simulink model "PubIfDecisionLSM_MDL"  (R2020b)
settings: configuration reference "DspaceConfig" (kept outside this file)
PostLoadFcn:
  | if any(exist('dsrtsu_mdlpostloadfcn', 'file') ~= 0), dsrtsu_mdlpostloadfcn('Execute', bdroot); end
InitFcn:
  | , if any(exist('rtifpga_mdlclblib', 'file') ~= 0), rtifpga_mdlclblib('Init', bdroot); end,
  | , if any(exist('dsmpb_private', 'file') ~= 0), dsmpb_private('dsmpb_mdlclblib', 'Init', bdroot); end,
values from neighbouring files (symbols this model uses):
  P_LSM_ALC_Enable = 0.0    [LSM_Parameter.sldd]
  P_LSM_AwayEdge_offset = 0.1    [LSM_Parameter.sldd]
  P_LSM_CentValidErr = 1.0    [LSM_Parameter.sldd]
  P_LSM_DOP_C0_EN_Limit = 0.8    [LSM_Parameter.sldd]
  P_LSM_DOP_C0_out_Limit = 2.0    [LSM_Parameter.sldd]
  P_LSM_DOP_C1_EN_Limit : value not decoded    [LSM_Parameter.sldd]
  P_LSM_DOP_C1_out_Limit : value not decoded    [LSM_Parameter.sldd]
  P_LSM_DOP_C1AndC2_Lim_X : value not decoded    [LSM_Parameter.sldd]
  P_LSM_DOP_C2_EN_Limit : value not decoded    [LSM_Parameter.sldd]
  P_LSM_DOP_C2_out_Limit : value not decoded    [LSM_Parameter.sldd]
  P_LSM_DOP_In_Pre2Dop_Dis = 1.0    [LSM_Parameter.sldd]
  P_LSM_DOP_Out_Pre2Dop_Dis = 2.0    [LSM_Parameter.sldd]
  P_LSM_DOP_PreDis_X : value not decoded    [LSM_Parameter.sldd]
  P_LSM_DOP_PreDis_Y : value not decoded    [LSM_Parameter.sldd]
  P_LSM_DOPEnableSW = 1.0    [LSM_Parameter.sldd]
  P_LSM_DOPValid_CheckTime = 0.06    [LSM_Parameter.sldd]
  P_LSM_DoubleLine_Curr2Cent_Dislimit = 0.5    [LSM_Parameter.sldd]
  P_LSM_DoubleLine_Dop2Cent_Dislimit = 0.5    [LSM_Parameter.sldd]
  P_LSM_DoubleLine_DOPOut_C1 : value not decoded    [LSM_Parameter.sldd]
  P_LSM_DoubleLine_Pre2Cent_Dislimit = 1.0    [LSM_Parameter.sldd]
  P_LSM_Error_Limit = 0.5    [LSM_Parameter.sldd]
  P_LSM_IFV2CenterAxis = 0.0    [LSM_Parameter.sldd]
  P_LSM_IFV2RearAxis = 0.0    [LSM_Parameter.sldd]
  P_LSM_Line2Edge_limit = 0.5    [LSM_Parameter.sldd]
  P_LSM_Line_Error = 0.1    [LSM_Parameter.sldd]
  P_LSM_LineSTD_Limit = 0.15    [LSM_Parameter.sldd]
  P_LSM_NOH_Switch = 0.0    [LSM_Parameter.sldd]
  P_LSM_OTL_C0_Factor = 1.0    [LSM_Parameter.sldd]
  P_LSM_OTL_C1_Factor = 0.5    [LSM_Parameter.sldd]
  P_LSM_OTL_C2_Factor = 0.5    [LSM_Parameter.sldd]
  P_LSM_Pre2OnlyLineDis = 5.0    [LSM_Parameter.sldd]
  P_LSM_Pre_t = 0.0    [LSM_Parameter.sldd]
  P_LSM_SingleLine_Cent2Edge_Dislimit = 100.0    [LSM_Parameter.sldd]
  P_LSM_SingleLine_Curr2Cent_Dislimit = 0.2    [LSM_Parameter.sldd]
  P_LSM_SingleLine_Dop2Cent_Dislimit = 0.2    [LSM_Parameter.sldd]
  P_LSM_SingleLine_DOPOut_C1 : value not decoded    [LSM_Parameter.sldd]
  P_LSM_SingleLine_Pre2Cent_Dislimit = 0.5    [LSM_Parameter.sldd]
  P_LSM_TJALimitSpd = 60.0    [LSM_Parameter.sldd]
undefined symbols (not defined in the file or in its folder): P_lCS_IFV2CenterAxis, P_LCS_IFV2RearAxis, P_LSM_EntryEdge_offset, P_LSM_EntryLnChngEnSwitch, P_LSM_EntryVanishDis, P_LSM_LinetLostTime, P_LSM_LineWijCal_C12, P_LSM_LineWijCal_C13, P_LSM_MapValid_ErrorSwitch, P_LSM_PosLineLcFac, P_LSM_SpdLim_Stub_Spd, P_LSM_SpdLim_StubLength, P_LSM_SpdTurnAlarm
libraries: simulink x324, TrueDurationTime x11
(part 11 of 25)

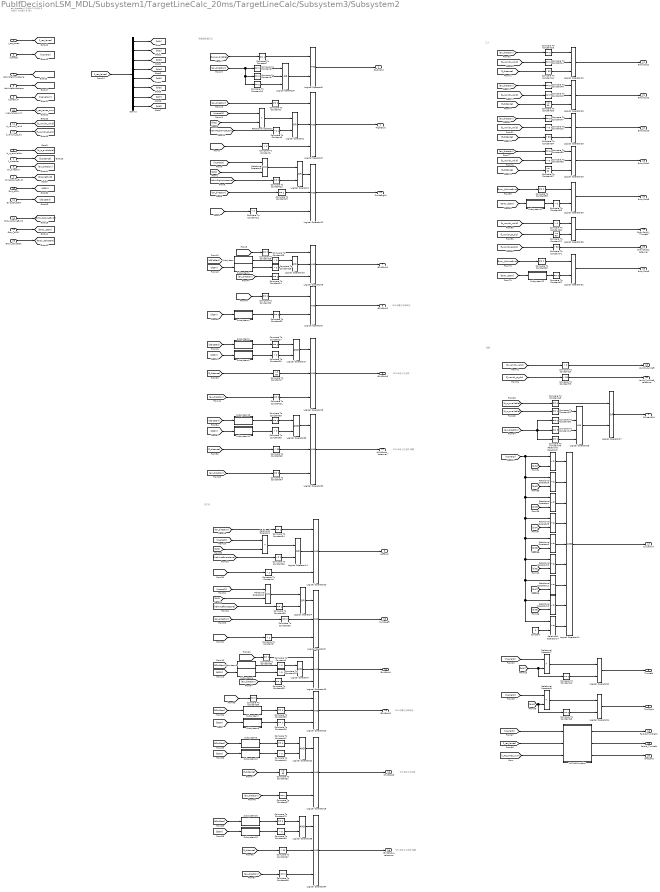
== system PubIfDecisionLSM_MDL/Subsystem1/TargetLineCalc_20ms/TargetLineCalc/Subsystem3/Subsystem2 ==
  note: 左汇出
  note: 巡航
  note: 汇入
  note: %%未走上汇出线
  note: %%沿着汇出线驶出
  note: %%未走上汇出线
  note: en_direction
      | 1 左驶出
      | 2 右驶出
      | 3 左直行
      | 4 右直行
      | 5 驶入
  note: %%沿着汇出线驶出
  note: 高速或匝道汇出
  note: %%未走上汇出线,接管
  note: %%未走上汇出线,接管
  Exit_bIsLineExist : Inport
  f_distance : Inport  Port=2
  b_is_available : Inport  Port=3
  i_rec_lanes : Inport  Port=4
  nLaneID : Inport  Port=5
  en_direction : Inport  Port=6
  VehInRightmostLane : Inport  Port=7  OutDataTypeStr=boolean
  VehInLeftmostLane : Inport  Port=8  OutDataTypeStr=boolean
  nLaneNum : Inport  Port=9
  i_rec_lanes_num : Inport  Port=10
  " b_vanish_valid" : Inport  Port=11
  " Exit_dDisStart" : Inport  Port=12
  Exit_dC0V : Inport  Port=13
  Entry_bIsLineExist : Inport  Port=14
  Entry_dDisStart : Inport  Port=15
  Entry_dC0V : Inport  Port=16
  " f_vanish_pt_dis " : Inport  Port=17
  Compare To Constant{1,4..5,12} (4 alike) : simulink/Logic and Bit Operations/Compare To Constant  relop=<  const=2  OutDataTypeStr=boolean
  Compare To Constant{10,16,46..47,56} (5 alike) : simulink/Logic and Bit Operations/Compare To Constant  relop===  const=5  OutDataTypeStr=boolean
  Compare To Constant11 : simulink/Logic and Bit Operations/Compare To Constant  relop===  const=3  OutDataTypeStr=boolean
  Compare To Constant{6,13,15,20,25..26,29,40,55,59,62,66,69} (13 alike) : simulink/Logic and Bit Operations/Compare To Constant  relop=>  const=0  OutDataTypeStr=boolean
  Compare To Constant{14,27..28,30,41,45,48,50,52,61,65,70} (12 alike) : simulink/Logic and Bit Operations/Compare To Constant  relop===  const=0  OutDataTypeStr=boolean
  Compare To Constant17 : simulink/Logic and Bit Operations/Compare To Constant  relop=>=  const=50  OutDataTypeStr=boolean
  Compare To Constant{2,9,18..19,21,23..24,32,38,58,60,64} (12 alike) : simulink/Logic and Bit Operations/Compare To Constant  relop===  const=2  OutDataTypeStr=boolean
  Compare To Constant{7..8,22,33..35,37,39,51,68} (10 alike) : simulink/Logic and Bit Operations/Compare To Constant  relop===  const=1  OutDataTypeStr=boolean
  Compare To Constant3 : simulink/Logic and Bit Operations/Compare To Constant  relop=~=  const=1  OutDataTypeStr=boolean
  Compare To Constant31 : simulink/Logic and Bit Operations/Compare To Constant  relop=>=  const=50  OutDataTypeStr=boolean
  Compare To Constant36 : simulink/Logic and Bit Operations/Compare To Constant  relop=~=  const=1  OutDataTypeStr=boolean
  Compare To Constant42 : simulink/Logic and Bit Operations/Compare To Constant  relop=~=  const=0  OutDataTypeStr=boolean
  Compare To Constant43 : simulink/Logic and Bit Operations/Compare To Constant  relop=~=  const=0  OutDataTypeStr=boolean
  Compare To Constant44 : simulink/Logic and Bit Operations/Compare To Constant  relop=>  const=50  OutDataTypeStr=boolean
  Compare To Constant49 : simulink/Logic and Bit Operations/Compare To Constant  relop===  const=4  OutDataTypeStr=boolean
  Compare To Constant53 : simulink/Logic and Bit Operations/Compare To Constant  relop=<=  const=50  OutDataTypeStr=boolean
  Compare To Constant54 : simulink/Logic and Bit Operations/Compare To Constant  relop=>  const=50  OutDataTypeStr=boolean
  Compare To Constant57 : simulink/Logic and Bit Operations/Compare To Constant  relop=<=  const=50  OutDataTypeStr=boolean
  Compare To Constant{63,67,71,73} (4 alike) : simulink/Logic and Bit Operations/Compare To Constant  relop=<  const=50  OutDataTypeStr=boolean
  Compare To Constant72 : simulink/Logic and Bit Operations/Compare To Constant  relop=>=  const=50  OutDataTypeStr=boolean
  Constant : Constant  Value=0  OutDataTypeStr=uint8
  Demux : Demux  Outputs=8
  Logical Operator{1..2,4,14,27} (5 alike) : Logic  Operator=OR  AllPortsSameDT=off  OutDataTypeStr=boolean
  Logical Operator{3,5,10,12..13,15,18..20,23,25..26,29,32,34} (15 alike) : Logic  Inputs=3  AllPortsSameDT=off  OutDataTypeStr=boolean
  Logical Operator11 : Logic  Inputs=9'  AllPortsSameDT=off  OutDataTypeStr=boolean
  Logical Operator{6..8,16..17,21..22,24,30..31,33,35..36} (13 alike) : Logic  AllPortsSameDT=off  OutDataTypeStr=boolean
  Logical Operator28 : Logic  Inputs=4  AllPortsSameDT=off  OutDataTypeStr=boolean
  Logical Operator9 : Logic  Operator=OR  Inputs=3  AllPortsSameDT=off  OutDataTypeStr=boolean
  MATLAB Function : MATLAB Function  TreatAsAtomicUnit=on
  Relational Operator : RelationalOperator  Operator=<  OutDataTypeStr=boolean  RndMeth=Simplest
  Relational Operator1 : RelationalOperator  Operator=>  OutDataTypeStr=boolean  RndMeth=Simplest
  Relational Operator{2..6,10,12..14} (9 alike) : RelationalOperator  Operator=~=  OutDataTypeStr=boolean  RndMeth=Simplest
  Relational Operator11 : RelationalOperator  Operator===  OutDataTypeStr=boolean  RndMeth=Simplest
  Relational Operator7 : RelationalOperator  Operator=>  OutDataTypeStr=boolean  RndMeth=Simplest
  Relational Operator8 : RelationalOperator  Operator=<  OutDataTypeStr=boolean  RndMeth=Simplest
  Relational Operator9 : RelationalOperator  Operator===  OutDataTypeStr=boolean  RndMeth=Simplest
  Subsystem : Subsystem
  Subsystem1 : Subsystem
  Subsystem10 : Subsystem
  Subsystem11 : Subsystem
  Subsystem12 : Subsystem
  Subsystem13 : Subsystem
  Subsystem14 : Subsystem
  Subsystem15 : Subsystem
  Subsystem16 : Subsystem
  Subsystem2 : Subsystem
  Subsystem3 : Subsystem
  Subsystem4 : Subsystem
  Subsystem5 : Subsystem
  Subsystem6 : Subsystem
  Subsystem7 : Subsystem
  Subsystem8 : Subsystem
  Subsystem9 : Subsystem
  StubValid : Outport
  RightStub : Outport  Port=2
  LeftStub : Outport  Port=3
  CruiseValid : Outport  Port=4
  TurnLeft : Outport  Port=5
  TurnRight : Outport  Port=6
  rExitStub1 : Outport  Port=7
  rExitStub2 : Outport  Port=8
  rExitStub3 : Outport  Port=9
  Vanish_turnleft : Outport  Port=10
  EntryStub1 : Outport  Port=11
  CruiseRight : Outport  Port=12
  CruiseLeft : Outport  Port=13
  lExitStub1 : Outport  Port=14
  lExitStub2 : Outport  Port=15
  lExitStub3 : Outport  Port=16
  CruiseTurn : Outport  Port=17
  Forbid_TurnRight : Outport  Port=18
  Forbid_TurnLeft : Outport  Port=19
  OneLane : Outport  Port=20
  EntryStub2 : Outport  Port=21
  EntryStub3 : Outport  Port=22
  EntryStub4 : Outport  Port=23
  EntryStub5 : Outport  Port=24
  EntryStub6 : Outport  Port=25
  EntryStub5_TurnLeft : Outport  Port=26
  rExitStub4_takeover : Outport  Port=27
  lExitStub4_takeover : Outport  Port=28
  EntryStub5_takeover : Outport  Port=29
  Vanish_turnleft_takeover : Outport  Port=30
  wires:
  Compare To Constant40/1 -> Logical Operator22/2
  Compare To Constant41/1 -> Logical Operator22/1
  Subsystem9/1(y) -> Compare To Constant41/1
  [dDisStart] -> Subsystem9/1(u)
  [dC0V] -> Subsystem10/1(u)
  Subsystem10/1(y) -> Compare To Constant40/1
  Subsystem8/1(y) -> Compare To Constant28/1
  [dC0V] -> Subsystem8/1(u)
  [dDisStart] -> Subsystem7/1(u)
  Subsystem7/1(y) -> Compare To Constant30/1
  Compare To Constant30/1 -> Logical Operator23/2
  Compare To Constant28/1 -> Logical Operator23/3
  Logical Operator7/1 -> Logical Operator19/2
  Compare To Constant13/1 -> Logical Operator7/2
  Compare To Constant6/1 -> Logical Operator7/1
  Subsystem5/1(y) -> Compare To Constant6/1
  [dDisStart] -> Subsystem5/1(u)
  [dC0V] -> Subsystem6/1(u)
  Subsystem6/1(y) -> Compare To Constant13/1
  Subsystem3/1(y) -> Compare To Constant29/1
  [dC0V] -> Subsystem3/1(u)
  [dDisStart] -> Subsystem2/1(u)
  Subsystem2/1(y) -> Compare To Constant27/1
  Compare To Constant27/1 -> Logical Operator17/1
  Compare To Constant29/1 -> Logical Operator17/2
  Compare To Constant52/1 -> Logical Operator6/2
  [dC0V] -> Subsystem4/1(u)
  Subsystem4/1(y) -> Compare To Constant52/1
  Subsystem1/1(y) -> Compare To Constant26/1
  [dC0V] -> Subsystem1/1(u)
  [dDisStart] -> Subsystem/1(u)
  [i_rec_lanes_num] -> MATLAB Function/3(i_rec_lanes_num)
  MATLAB Function/3(OneLane) -> OneLane/1
  MATLAB Function/2(Forbid_TurnLeft) -> Forbid_TurnLeft/1
  MATLAB Function/1(Forbid_TurnRight) -> Forbid_TurnRight/1
  [nLaneID] -> MATLAB Function/1(nLaneID)
  [i_rec_lanes] -> MATLAB Function/2(i_rec_lanes)
  Logical Operator27/1 -> CruiseValid/1  "CruiseValid"
  Compare To Constant49/1 -> Logical Operator28/4
  Compare To Constant51/1 -> Logical Operator28/1
  [b_is_available] -> Compare To Constant51/1
  [en_direction] -> Compare To Constant11/1, Compare To Constant49/1, Compare To Constant50/1
  Compare To Constant50/1 -> Logical Operator28/2
  Compare To Constant11/1 -> Logical Operator28/3
  Logical Operator28/1 -> Logical Operator27/2
  Constant/1 -> Relational Operator14/2
  Relational Operator14/1 -> Logical Operator11/9
  Compare To Constant12/1 -> Logical Operator12/3
  Logical Operator8/1 -> StubValid/1  "StubValid"
  Logical Operator9/1 -> Logical Operator8/2
  Compare To Constant10/1 -> Logical Operator9/3
  Compare To Constant9/1 -> Logical Operator9/2
  Compare To Constant8/1 -> Logical Operator9/1
  [en_direction] -> Compare To Constant8/1, Compare To Constant9/1, Compare To Constant10/1
  Relational Operator7/1 -> Logical Operator21/1
  [bit8] -> Relational Operator13/2
  [bit7] -> Relational Operator12/2
  [bit6] -> Relational Operator10/2
  Relational Operator13/1 -> Logical Operator11/8
  Relational Operator12/1 -> Logical Operator11/7
  Relational Operator10/1 -> Logical Operator11/6
  [b_is_available] -> Compare To Constant48/1
  Compare To Constant48/1 -> Logical Operator27/1
  Compare To Constant37/1 -> Logical Operator18/3
  Logical Operator19/1 -> lExitStub1/1  "lExitStub1"
  [en_direction] -> Compare To Constant37/1
  Compare To Constant39/1 -> Logical Operator19/3
  [f_distance] -> Compare To Constant31/1
  [en_direction] -> Compare To Constant39/1
  Logical Operator18/1 -> lExitStub3/1  "lExitStub3"
  Logical Operator22/1 -> Logical Operator18/1
  Compare To Constant31/1 -> Logical Operator18/2
  [bIsLineExist] -> Compare To Constant32/1
  Compare To Constant32/1 -> Logical Operator19/1
  Compare To Constant38/1 -> Logical Operator23/1
  [bIsLineExist] -> Compare To Constant38/1
  Logical Operator23/1 -> lExitStub2/1  "lExitStub2"
  Logical Operator20/1 -> LeftStub/1  "LeftStub"
  [en_direction] -> Compare To Constant33/1  "LSM_Stub_Direction"
  Relational Operator1/1 -> Logical Operator14/1
  [bit1] -> Relational Operator1/2
  Logical Operator5/1 -> CruiseLeft/1  "CruiseLeft"
  [VehInLeftmostLane] -> Compare To Constant36/1
  Relational Operator11/1 -> Logical Operator4/1
  [nLaneID] -> Relational Operator1/1
  [VehInLeftmostLane] -> Compare To Constant35/1
  Compare To Constant35/1 -> Logical Operator4/2
  Logical Operator4/1 -> Logical Operator5/1
  Compare To Constant33/1 -> Logical Operator5/2
  [en_direction] -> Compare To Constant34/1  "LSM_Stub_Direction"
  Compare To Constant34/1 -> Logical Operator20/1
  [nLaneID] -> Relational Operator11/1
  [bit1] -> Relational Operator11/2
  Compare To Constant5/1 -> Logical Operator5/3
  Logical Operator14/1 -> Logical Operator20/2
  [bIsLineExist] -> Compare To Constant5/1
  Compare To Constant4/1 -> Logical Operator20/3
  [bIsLineExist] -> Compare To Constant4/1
  Compare To Constant36/1 -> Logical Operator14/2
  Logical Operator6/1 -> rExitStub2/1  "rExitStub2"
  [bIsLineExist] -> Compare To Constant23/1
  Compare To Constant23/1 -> Logical Operator6/1
  Compare To Constant18/1 -> Logical Operator15/1
  [bIsLineExist] -> Compare To Constant18/1
  [bIsLineExist] -> Compare To Constant12/1
  Exit_bIsLineExist/1 -> [bIsLineExist]
  Compare To Constant1/1 -> Logical Operator3/3
  [bIsLineExist] -> Compare To Constant1/1
  [b_is_available] -> Compare To Constant7/1
  b_is_available/1 -> [b_is_available]
  Compare To Constant22/1 -> Logical Operator1/2
  [en_direction] -> Compare To Constant19/1  "LSM_Stub_Direction"
  [bit1] -> Relational Operator9/2
  Compare To Constant19/1 -> Logical Operator12/2
  Relational Operator9/1 -> Logical Operator1/1
  Logical Operator1/1 -> Logical Operator12/1
  Logical Operator12/1 -> CruiseRight/1  "CruiseRight"
  [VehInRightmostLane] -> Compare To Constant22/1
  [nLaneID] -> Relational Operator9/1
  Logical Operator10/1 -> EntryStub1/1  "EntryStub1"
  Logical Operator11/1 -> CruiseTurn/1  "CruiseTurn"
  Compare To Constant17/1 -> Logical Operator13/2
  VehInRightmostLane/1 -> [VehInRightmostLane]
  " Exit_dDisStart"/1 -> [dDisStart]
  nLaneID/1 -> [nLaneID]
  VehInLeftmostLane/1 -> [VehInLeftmostLane]
  f_distance/1 -> [f_distance]
  [en_direction] -> Compare To Constant2/1  "LSM_Stub_Direction"
  Relational Operator2/1 -> Logical Operator11/1
  Relational Operator4/1 -> Logical Operator11/3
  [bit1] -> Relational Operator2/2
  [bit1] -> Compare To Constant43/1, Relational Operator8/2
  [nLaneID] -> Relational Operator8/1
  Relational Operator8/1 -> Logical Operator24/1
  [nLaneID] -> Relational Operator/1
  [bit1] -> Compare To Constant42/1, Relational Operator7/2
  [en_direction] -> Compare To Constant16/1  "LSM_Stub_Direction"
  Logical Operator17/1 -> Logical Operator13/1
  nLaneNum/1 -> [nLaneNum]
  i_rec_lanes_num/1 -> [i_rec_lanes_num]
  [b_vanish_valid] -> Compare To Constant14/1
  Compare To Constant20/1 -> Vanish_turnleft/1  "Vanish_turnleft"
  Subsystem/1(y) -> Compare To Constant25/1
  Logical Operator3/1 -> RightStub/1  "RightStub"
  Logical Operator16/1 -> Logical Operator15/2
  [bit1] -> Relational Operator/2
  [bit2] -> Relational Operator3/2
  [bit3] -> Relational Operator4/2
  Compare To Constant14/1 -> Logical Operator10/2
  [bit5] -> Relational Operator6/2
  Exit_dC0V/1 -> [dC0V]
  [VehInRightmostLane] -> Compare To Constant3/1
  Compare To Constant7/1 -> Logical Operator8/1
  Logical Operator13/1 -> rExitStub3/1  "rExitStub3"
  " b_vanish_valid"/1 -> [b_vanish_valid]
  [en_direction] -> Compare To Constant24/1
  [bit4] -> Relational Operator5/2
  Compare To Constant2/1 -> Logical Operator3/1
  Logical Operator2/1 -> Logical Operator3/2
  Relational Operator/1 -> Logical Operator2/1
  Compare To Constant16/1 -> Logical Operator10/1
  [b_vanish_valid] -> Compare To Constant20/1
  [f_distance] -> Compare To Constant17/1
  Relational Operator6/1 -> Logical Operator11/5
  [nLaneID] -> Relational Operator2/1, Relational Operator6/1, Relational Operator13/1, Relational Operator14/1, Relational Operator12/1, Relational Operator10/1, Relational Operator5/1, Relational Operator4/1, Relational Operator3/1
  en_direction/1 -> [en_direction]
  Compare To Constant24/1 -> Logical Operator15/3
  Compare To Constant25/1 -> Logical Operator16/1
  [en_direction] -> Compare To Constant21/1
  Logical Operator15/1 -> rExitStub1/1  "rExitStub1"
  Relational Operator3/1 -> Logical Operator11/2
  Compare To Constant26/1 -> Logical Operator16/2
  Relational Operator5/1 -> Logical Operator11/4
  [nLaneID] -> Relational Operator7/1
  Compare To Constant3/1 -> Logical Operator2/2
  Compare To Constant21/1 -> Logical Operator13/3
  Compare To Constant42/1 -> Logical Operator21/2
  Logical Operator21/1 -> TurnLeft/1  "TurnLeft"
  Compare To Constant43/1 -> Logical Operator24/2
  Logical Operator24/1 -> TurnRight/1  "TurnLeft"
  [i_rec_lanes] -> Demux/1
  Demux/5 -> [bit5]
  Demux/4 -> [bit4]
  Demux/6 -> [bit6]
  Demux/7 -> [bit7]
  Demux/8 -> [bit8]
  Demux/1 -> [bit1]
  Demux/3 -> [bit3]
  Demux/2 -> [bit2]
  i_rec_lanes/1 -> [i_rec_lanes]
  Entry_dC0V/1 -> [Entry_dC0V]
  Entry_dDisStart/1 -> [Entry_dDisStart]
  Entry_bIsLineExist/1 -> [Entry_bIsLineExist]
  [f_distance] -> Compare To Constant44/1
  Compare To Constant44/1 -> Logical Operator10/3
  Compare To Constant53/1 -> Logical Operator26/3
  [f_distance] -> Compare To Constant53/1
  Compare To Constant46/1 -> Logical Operator26/1
  Compare To Constant45/1 -> Logical Operator26/2
  [b_vanish_valid] -> Compare To Constant45/1
  [en_direction] -> Compare To Constant46/1  "LSM_Stub_Direction"
  Logical Operator26/1 -> EntryStub2/1  "EntryStub2"
  Logical Operator29/1 -> EntryStub4/1  "EntryStub4"
  [en_direction] -> Compare To Constant56/1  "LSM_Stub_Direction"
  [b_vanish_valid] -> Compare To Constant55/1
  Compare To Constant55/1 -> Logical Operator29/2
  Compare To Constant56/1 -> Logical Operator29/1
  [f_distance] -> Compare To Constant57/1
  Compare To Constant57/1 -> Logical Operator29/3
  Compare To Constant54/1 -> Logical Operator25/3
  [f_distance] -> Compare To Constant54/1
  Compare To Constant47/1 -> Logical Operator25/1
  Compare To Constant15/1 -> Logical Operator25/2
  [b_vanish_valid] -> Compare To Constant15/1
  [en_direction] -> Compare To Constant47/1  "LSM_Stub_Direction"
  Logical Operator25/1 -> EntryStub3/1  "EntryStub3"
  [Entry_bIsLineExist] -> Compare To Constant58/1
  Compare To Constant58/1 -> Logical Operator30/1
  [Entry_dC0V] -> Subsystem11/1(u)
  Subsystem11/1(y) -> Compare To Constant59/1
  Compare To Constant59/1 -> Logical Operator30/2
  Logical Operator30/1 -> EntryStub5/1  "EntryStub5"
  Logical Operator31/1 -> EntryStub6/1  "EntryStub6"
  Compare To Constant61/1 -> Logical Operator31/2
  Subsystem12/1(y) -> Compare To Constant61/1
  [Entry_dC0V] -> Subsystem12/1(u)
  Compare To Constant60/1 -> Logical Operator31/1
  [Entry_bIsLineExist] -> Compare To Constant60/1
  Compare To Constant62/1 -> Logical Operator36/1
  [b_vanish_valid] -> Compare To Constant62/1
  Compare To Constant64/1 -> Logical Operator32/3
  [en_direction] -> Compare To Constant64/1
  [f_distance] -> Compare To Constant63/1
  Logical Operator32/1 -> rExitStub4_takeover/1  "rExitStub4_takeover"
  Logical Operator33/1 -> Logical Operator32/1
  Compare To Constant63/1 -> Logical Operator32/2
  Compare To Constant66/1 -> Logical Operator33/2
  Compare To Constant65/1 -> Logical Operator33/1
  Subsystem13/1(y) -> Compare To Constant65/1
  [dDisStart] -> Subsystem13/1(u)
  [dC0V] -> Subsystem14/1(u)
  Subsystem14/1(y) -> Compare To Constant66/1
  Compare To Constant67/1 -> Logical Operator34/2
  Logical Operator35/1 -> Logical Operator34/1
  Logical Operator34/1 -> lExitStub4_takeover/1  "lExitStub4_takeover"
  [f_distance] -> Compare To Constant67/1
  [en_direction] -> Compare To Constant68/1
  Compare To Constant68/1 -> Logical Operator34/3
  Subsystem15/1(y) -> Compare To Constant69/1
  [dC0V] -> Subsystem15/1(u)
  [dDisStart] -> Subsystem16/1(u)
  Subsystem16/1(y) -> Compare To Constant70/1
  Compare To Constant70/1 -> Logical Operator35/1
  Compare To Constant69/1 -> Logical Operator35/2
  [f_vanish_pt_dis] -> Compare To Constant71/1
  Compare To Constant71/1 -> EntryStub5_takeover/1  "EntryStub5_takeover"
  " f_vanish_pt_dis "/1 -> [f_vanish_pt_dis]
  [f_vanish_pt_dis] -> Compare To Constant72/1
  Compare To Constant72/1 -> Logical Operator36/2
  Logical Operator36/1 -> EntryStub5_TurnLeft/1  "EntryStub5_TurnLeft"
  [f_vanish_pt_dis] -> Compare To Constant73/1
  Compare To Constant73/1 -> Vanish_turnleft_takeover/1  "Vanish_turnleft_takeover"

== system PubIfDecisionLSM_MDL/Subsystem1/TargetLineCalc_20ms/TargetLineCalc/Subsystem3/Subsystem3 ==
  PilotTurnSwSts : Inport
  nLaneID : Inport  Port=2
  Compare To Constant2 : simulink/Logic and Bit Operations/Compare To Constant  relop===  const=1  OutDataTypeStr=boolean
  Compare To Constant3 : simulink/Logic and Bit Operations/Compare To Constant  relop===  const=2  OutDataTypeStr=boolean
  Constant : Constant  OutDataTypeStr=uint8
  Constant1 : Constant  Value=2  OutDataTypeStr=uint8
  Constant2 : Constant  Value=0  OutDataTypeStr=uint8
  Logical Operator1 : Logic  AllPortsSameDT=off  OutDataTypeStr=boolean
  Logical Operator2 : Logic  AllPortsSameDT=off  OutDataTypeStr=boolean
  Relational Operator1 : RelationalOperator  Operator=<  OutDataTypeStr=boolean  RndMeth=Simplest
  Relational Operator2 : RelationalOperator  Operator=>  OutDataTypeStr=boolean  RndMeth=Simplest
  Switch : Switch  Criteria=u2 > Threshold
  Switch1 : Switch  Criteria=u2 > Threshold
  Unit Delay{,1..3} (4 alike) : UnitDelay  SampleTime=-1  HasFrameUpgradeWarning=on
  LaneChange : Outport
  wires:
  Relational Operator1/1 -> Logical Operator1/2
  Compare To Constant2/1 -> Logical Operator1/1
  Constant/1 -> Switch/1
  Constant2/1 -> Switch1/3
  Unit Delay2/1 -> Compare To Constant3/1
  Logical Operator1/1 -> Switch/2
  Unit Delay/1 -> Relational Operator1/2
  PilotTurnSwSts/1 -> Unit Delay2/1, Unit Delay3/1
  Logical Operator2/1 -> Switch1/2
  Unit Delay3/1 -> Compare To Constant2/1
  Constant1/1 -> Switch1/1
  Unit Delay1/1 -> Relational Operator2/2
  Compare To Constant3/1 -> Logical Operator2/1
  Switch1/1 -> Switch/3
  nLaneID/1 -> Relational Operator2/1, Unit Delay1/1, Unit Delay/1, Relational Operator1/1
  Relational Operator2/1 -> Logical Operator2/2
  Switch/1 -> LaneChange/1  "LaneChange"

== system PubIfDecisionLSM_MDL/Subsystem1/TargetLineCalc_20ms/TargetLineCalc/Subsystem4/If Action Subsystem ==
  In1 : Inport
  Action Port : ActionPort  ActionPortLabel=if(u1 > 0)
  LH1Wij : Outport
  wires:
  In1/1 -> LH1Wij/1

== system PubIfDecisionLSM_MDL/Subsystem1/TargetLineCalc_20ms/TargetLineCalc/Subsystem4/If Action Subsystem1 ==
  In1 : Inport
  Action Port : ActionPort  ActionPortLabel=if(u1 > 0)
  LH1Wij : Outport
  wires:
  In1/1 -> LH1Wij/1

== system PubIfDecisionLSM_MDL/Subsystem1/TargetLineCalc_20ms/TargetLineCalc/Subsystem4/If Action Subsystem2 ==
  Action Port : ActionPort  ActionPortLabel=else
  Constant : Constant  Value=0  OutDataTypeStr=single
  LH1Wij : Outport
  wires:
  Constant/1 -> LH1Wij/1

== system PubIfDecisionLSM_MDL/Subsystem1/TargetLineCalc_20ms/TargetLineCalc/Subsystem4/If Action Subsystem3 ==
  Action Port : ActionPort  ActionPortLabel=else
  Constant : Constant  Value=0  OutDataTypeStr=single
  LH1Wij : Outport
  wires:
  Constant/1 -> LH1Wij/1

== system PubIfDecisionLSM_MDL/Subsystem1/TargetLineCalc_20ms/TargetLineCalc/Subsystem4/If Action Subsystem4 ==
  In1 : Inport
  In2 : Inport  Port=2
  Action Port : ActionPort  ActionPortLabel=else
  Out1 : Outport
  Out2 : Outport  Port=2
  wires:
  In1/1 -> Out1/1
  In2/1 -> Out2/1

== system PubIfDecisionLSM_MDL/Subsystem1/TargetLineCalc_20ms/TargetLineCalc/Subsystem4/If Action Subsystem5 ==
  Action Port : ActionPort  ActionPortLabel=if(u1 > 0)
  Constant : Constant  Value=P_LSM_PosLineLcFac
  Out1 : Outport
  Out2 : Outport  Port=2
  wires:
  Constant/1 -> Out2/1, Out1/1

== system PubIfDecisionLSM_MDL/Subsystem1/TargetLineCalc_20ms/TargetLineCalc/Subsystem5/If Action Subsystem ==
  In1 : Inport
  Action Port : ActionPort  ActionPortLabel=if(u1 > 0)
  LH1Wij : Outport
  wires:
  In1/1 -> LH1Wij/1

== system PubIfDecisionLSM_MDL/Subsystem1/TargetLineCalc_20ms/TargetLineCalc/Subsystem5/If Action Subsystem1 ==
  In1 : Inport
  Action Port : ActionPort  ActionPortLabel=if(u1 > 0)
  LH1Wij : Outport
  wires:
  In1/1 -> LH1Wij/1

== system PubIfDecisionLSM_MDL/Subsystem1/TargetLineCalc_20ms/TargetLineCalc/Subsystem5/If Action Subsystem2 ==
  Action Port : ActionPort  ActionPortLabel=else
  Constant : Constant  Value=0  OutDataTypeStr=single
  LH1Wij : Outport
  wires:
  Constant/1 -> LH1Wij/1

== system PubIfDecisionLSM_MDL/Subsystem1/TargetLineCalc_20ms/TargetLineCalc/Subsystem5/If Action Subsystem3 ==
  Action Port : ActionPort  ActionPortLabel=else
  Constant : Constant  Value=0  OutDataTypeStr=single
  LH1Wij : Outport
  wires:
  Constant/1 -> LH1Wij/1

== system PubIfDecisionLSM_MDL/Subsystem1/TargetLineCalc_20ms/TargetLineCalc/Subsystem5/If Action Subsystem4 ==
  In1 : Inport
  In2 : Inport  Port=2
  Action Port : ActionPort  ActionPortLabel=else
  Out1 : Outport
  Out2 : Outport  Port=2
  wires:
  In1/1 -> Out1/1
  In2/1 -> Out2/1

== system PubIfDecisionLSM_MDL/Subsystem1/TargetLineCalc_20ms/TargetLineCalc/Subsystem5/If Action Subsystem5 ==
  Action Port : ActionPort  ActionPortLabel=if(u1 > 0)
  Constant : Constant  Value=P_LSM_PosLineLcFac
  Out1 : Outport
  Out2 : Outport  Port=2
  wires:
  Constant/1 -> Out2/1, Out1/1

== system PubIfDecisionLSM_MDL/Subsystem1/TargetLineCalc_20ms2/TargetLineCalc/Subsystem2/Subsystem1 ==
  "Input " : Inport
  Add : Sum  Inputs=+++++
  Add{1..5} (5 alike) : Sum  Inputs=+-
  Gain1 : Gain  Gain=1/5  OutDataTypeStr=single
  Gain{2..6} (5 alike) : Gain  Gain=1/0.02  OutDataTypeStr=single
  Unit Delay{,1..4} (5 alike) : UnitDelay  SampleTime=-1  HasFrameUpgradeWarning=on
  dInput : Outport
  wires:
  Gain6/1 -> Add/5
  Unit Delay4/1 -> Add5/2
  Add5/1 -> Gain6/1
  Gain5/1 -> Add/4
  Gain4/1 -> Add/3
  Gain3/1 -> Add/2
  Gain2/1 -> Add/1
  Add4/1 -> Gain5/1
  Add3/1 -> Gain4/1
  Add2/1 -> Gain3/1
  Unit Delay3/1 -> Add4/2, Add5/1, Unit Delay4/1
  Add1/1 -> Gain2/1
  Unit Delay2/1 -> Unit Delay3/1, Add3/2, Add4/1
  Unit Delay1/1 -> Add2/2, Add3/1, Unit Delay2/1
  Gain1/1 -> dInput/1
  "Input "/1 -> Unit Delay/1, Add1/1
  Unit Delay/1 -> Unit Delay1/1, Add1/2, Add2/1
  Add/1 -> Gain1/1

== system PubIfDecisionLSM_MDL/Subsystem1/TargetLineCalc_20ms2/TargetLineCalc/Subsystem2/Subsystem2 ==
  "Input " : Inport
  Add : Sum  Inputs=+++++
  Add{1..5} (5 alike) : Sum  Inputs=+-
  Gain1 : Gain  Gain=1/5  OutDataTypeStr=single
  Gain{2..6} (5 alike) : Gain  Gain=1/0.02  OutDataTypeStr=single
  Unit Delay{,1..4} (5 alike) : UnitDelay  SampleTime=-1  HasFrameUpgradeWarning=on
  dInput : Outport
  wires:
  Gain6/1 -> Add/5
  Unit Delay4/1 -> Add5/2
  Add5/1 -> Gain6/1
  Gain5/1 -> Add/4
  Gain4/1 -> Add/3
  Gain3/1 -> Add/2
  Gain2/1 -> Add/1
  Add4/1 -> Gain5/1
  Add3/1 -> Gain4/1
  Add2/1 -> Gain3/1
  Unit Delay3/1 -> Add4/2, Add5/1, Unit Delay4/1
  Add1/1 -> Gain2/1
  Unit Delay2/1 -> Unit Delay3/1, Add3/2, Add4/1
  Unit Delay1/1 -> Add2/2, Add3/1, Unit Delay2/1
  Gain1/1 -> dInput/1
  "Input "/1 -> Unit Delay/1, Add1/1
  Unit Delay/1 -> Unit Delay1/1, Add1/2, Add2/1
  Add/1 -> Gain1/1

== system PubIfDecisionLSM_MDL/Subsystem1/TargetLineCalc_20ms2/TargetLineCalc/Subsystem2/Subsystem3 ==
  "Input " : Inport
  Add : Sum  Inputs=+++++
  Add{1..5} (5 alike) : Sum  Inputs=+-
  Gain1 : Gain  Gain=1/5  OutDataTypeStr=single
  Gain{2..6} (5 alike) : Gain  Gain=1/0.02  OutDataTypeStr=single
  Unit Delay{,1..4} (5 alike) : UnitDelay  SampleTime=-1  HasFrameUpgradeWarning=on
  dInput : Outport
  wires:
  Add/1 -> Gain1/1
  Unit Delay/1 -> Add2/1, Add1/2, Unit Delay1/1
  "Input "/1 -> Add1/1, Unit Delay/1
  Gain1/1 -> dInput/1
  Unit Delay1/1 -> Unit Delay2/1, Add3/1, Add2/2
  Unit Delay2/1 -> Add4/1, Add3/2, Unit Delay3/1
  Add1/1 -> Gain2/1
  Unit Delay3/1 -> Unit Delay4/1, Add5/1, Add4/2
  Add2/1 -> Gain3/1
  Add3/1 -> Gain4/1
  Add4/1 -> Gain5/1
  Gain2/1 -> Add/1
  Gain3/1 -> Add/2
  Gain4/1 -> Add/3
  Gain5/1 -> Add/4
  Add5/1 -> Gain6/1
  Unit Delay4/1 -> Add5/2
  Gain6/1 -> Add/5

== system PubIfDecisionLSM_MDL/Subsystem1/TargetLineCalc_20ms2/TargetLineCalc/Subsystem3/EgoLineRef ==
  KapTraj : Inport
  VxvRef : Inport  Port=2
  TarLineValid : Inport  Port=3
  TarLineA3 : Inport  Port=4
  TarLineA2 : Inport  Port=5
  TarLineA1 : Inport  Port=6
  TarLineA0 : Inport  Port=7
  CalcEgoVehMove : MATLAB Function  TreatAsAtomicUnit=on
  CalcEgoVehMove1 : MATLAB Function  TreatAsAtomicUnit=on
  Compare To Constant93 : simulink/Logic and Bit Operations/Compare To Constant  relop=>  const=1  OutDataTypeStr=boolean
  Constant7 : Constant  Value=0.02  OutDataTypeStr=single
  Memory1 : Memory  InitialCondition=zeros(24,1)  InheritSampleTime=on
  Memory2 : Memory  InitialCondition=zeros(24,1)  InheritSampleTime=on
  Memory3 : Memory  InitialCondition=uint8(0)  InheritSampleTime=on
  Memory32 : Memory  InitialCondition=zeros(24,1)  InheritSampleTime=on
  Memory33 : Memory  InitialCondition=uint8(0)  InheritSampleTime=on
  Memory4 : Memory  InitialCondition=false  InheritSampleTime=on
  P0TrajHistCalc01 : MATLAB Function  TreatAsAtomicUnit=on
  Terminator{,1..6} (7 alike) : Terminator
  LaneChangeEnable : Outport
  wires:
  Compare To Constant93/1 -> CalcEgoVehMove1/4(TarLineValid)
  CalcEgoVehMove1/7(DxMin) -> Terminator6/1
  CalcEgoVehMove1/6(DxMax) -> Terminator5/1
  CalcEgoVehMove1/5(A0) -> Terminator4/1
  CalcEgoVehMove1/4(A1) -> Terminator3/1  "SinOfPsi"
  CalcEgoVehMove1/3(A2) -> Terminator2/1  "CosOfPsi"
  CalcEgoVehMove1/2(A3) -> Terminator1/1  "dDeltaY"
  CalcEgoVehMove1/1(EgoLineValid) -> Terminator/1  "dDeltaX"
  TarLineA0/1 -> CalcEgoVehMove1/8(TarLineA0)
  TarLineA1/1 -> CalcEgoVehMove1/7(TarLineA1)
  TarLineA2/1 -> CalcEgoVehMove1/6(TarLineA2)
  TarLineA3/1 -> CalcEgoVehMove1/5(TarLineA3)
  TarLineValid/1 -> Compare To Constant93/1
  Memory4/1 -> CalcEgoVehMove1/9(LaneChangeEnableK1)
  CalcEgoVehMove1/8(LaneChangeEnable) -> Memory4/1, LaneChangeEnable/1  "LSM_EnLaneChangeEnable"
  P0TrajHistCalc01/3(TrajHistDyv) -> CalcEgoVehMove1/3(Dyv), Memory1/1
  CalcEgoVehMove/4(SinOfPsi) -> P0TrajHistCalc01/4(EgoSinOfPsi)  "SinOfPsi"
  CalcEgoVehMove/3(CosOfPsi) -> P0TrajHistCalc01/3(EgoCosOfPsi)  "CosOfPsi"
  CalcEgoVehMove/2(dDeltaY) -> P0TrajHistCalc01/2(EgoDDeltaY)  "dDeltaY"
  CalcEgoVehMove/1(dDeltaX) -> P0TrajHistCalc01/1(EgoDDeltaX)  "dDeltaX"
  Memory3/1 -> P0TrajHistCalc01/9(CntK1)
  Memory2/1 -> P0TrajHistCalc01/8(TimeK1)
  P0TrajHistCalc01/4(Time) -> Memory2/1
  P0TrajHistCalc01/5(Cnt) -> Memory3/1
  P0TrajHistCalc01/2(TrajHistDxv) -> CalcEgoVehMove1/2(Dxv), Memory32/1
  Memory1/1 -> P0TrajHistCalc01/7(TrajHistDyvK1)
  Memory32/1 -> P0TrajHistCalc01/6(TrajHistDxvK1)
  P0TrajHistCalc01/1(TrajHistNum) -> CalcEgoVehMove1/1(Index), Memory33/1
  Memory33/1 -> P0TrajHistCalc01/5(TrajHistNumK1)
  KapTraj/1 -> CalcEgoVehMove/2(Kap)
  Constant7/1 -> CalcEgoVehMove/1(tCycle)
  VxvRef/1 -> CalcEgoVehMove/3(Vego)
